simulink model "ABS_fuzzy"  (R2017b)
settings: Solver=VariableStepAuto  StartTime=0.0  StopTime=60  RelTol=1e-3
InitFcn:
  | T_B = 0.1;
  | J = 1.13;
  | g = 9.81;
  | 
  | road_coeff = [
  |                 1.2801 23.990 0.5200
  |                 0.8570 33.822 0.3470
  |                 1.1973 25.168 0.5373
  |                 0.4004 33.708 0.1204
  |                 0.1946 94.129 0.0646
  |                 0.0500 306.39 0.0010
  |               ];
  | load('ANFIS.mat','train_fis');
  | ce = road_coeff(sel,:);
  | run controller_fis
undefined symbols (not defined in the file or in its folder): m, R, v_x
libraries: fuzblock x2, simulink x1
settings Model: Creator=hadlaczkyb  LastModifiedBy=hadlaczkyb

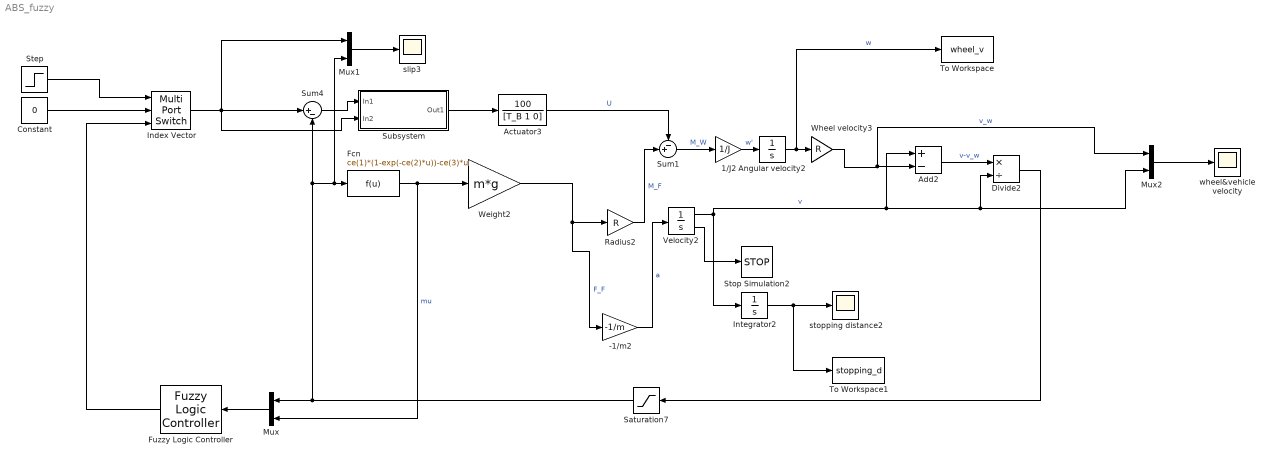
== system ABS_fuzzy ==
  -1/m2 : Gain  Gain=-1/m
  1/J2 : Gain  Gain=1/J
  Actuator3 : TransferFcn  Numerator=[0 0 100]  Denominator=[T_B 1 0]
  Add2 : Sum  Inputs=+-
  Angular velocity2 : Integrator  InitialCondition=v_x/R  LimitOutput=on  UpperSaturationLimit=1000  LowerSaturationLimit=0
  Constant : Constant  Value=0
  Divide2 : Product  Inputs=*/
  Fcn : Fcn  Expr=ce(1)*(1-exp(-ce(2)*u))-ce(3)*u
  Fuzzy Logic Controller : fuzblock/Fuzzy Logic  Controller  FIS=train_fis  OutputSampleNumber=101  DataType=double  FuzzifiedInputs=off  RuleFiringStrengths=off  RuleOutputs=off  AggregatedOutputs=off  SimulateUsing=Interpreted execution
  Index Vector : MultiPortSwitch  DataPortOrder=Zero-based contiguous  Inputs=2  zeroidx=on
  Integrator2 : Integrator
  Mux : Mux  Inputs=2
  Mux1 : Mux  Inputs=2
  Mux2 : Mux  Inputs=2
  Radius2 : Gain  Gain=R
  Saturation7 : Saturate  UpperLimit=1  LowerLimit=0
  Step : Step  Time=5  SampleTime=0
  Stop Simulation2 : Stop
  Subsystem : Subsystem
  Sum1 : Sum  Inputs=-+|
  Sum4 : Sum  Inputs=|+-
  To Workspace : ToWorkspace  VariableName=wheel_v  SaveFormat=Timeseries  SampleTime=-1
  To Workspace1 : ToWorkspace  VariableName=stopping_d  SaveFormat=Timeseries  SampleTime=-1
  Velocity2 : Integrator  InitialCondition=v_x  LimitOutput=on  UpperSaturationLimit=1000  LowerSaturationLimit=1  ShowSaturationPort=on
  Weight2 : Gain  Gain=m*g
  Wheel velocity3 : Gain  Gain=R
  slip3 : Scope
  stopping distance2 : Scope
  wheel&vehicle velocity : Scope
  wires:
  Sum4/1 -> Subsystem/1(In1)
  Mux/1 -> Fuzzy Logic Controller/1
  Saturation7/1 -> Mux1/2, Fcn/1, Sum4/2, Mux/1
  Mux1/1 -> slip3/1
  Fuzzy Logic Controller/1 -> Index Vector/3
  Subsystem/1(Out1) -> Actuator3/1
  Sum1/1 -> 1/J2/1  "M_W"
  -1/m2/1 -> Velocity2/1  "a"
  1/J2/1 -> Angular velocity2/1  "w'"
  Weight2/1 -> -1/m2/1, Radius2/1  "F_F"
  Velocity2/1 -> Integrator2/1, Divide2/2, Mux2/2, Add2/1  "v"
  Integrator2/1 -> To Workspace1/1, stopping distance2/1
  Fcn/1 -> Weight2/1, Mux/2  "mu"
  Divide2/1 -> Saturation7/1
  Radius2/1 -> Sum1/2  "M_F"
  Angular velocity2/1 -> To Workspace/1, Wheel velocity3/1  "w"
  Add2/1 -> Divide2/1  "v-v_w"
  Wheel velocity3/1 -> Add2/2, Mux2/1  "v_w"
  Velocity2/2 -> Stop Simulation2/1
  Actuator3/1 -> Sum1/1  "U"
  Mux2/1 -> wheel&vehicle velocity/1
  Step/1 -> Index Vector/1
  Constant/1 -> Index Vector/2
  Index Vector/1 -> Subsystem/2(In2), Sum4/1, Mux1/1

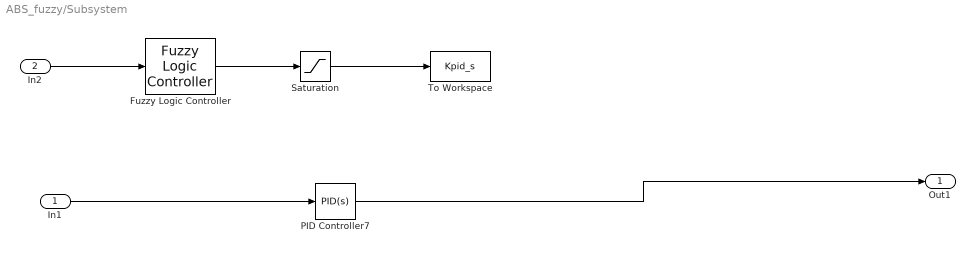
== system ABS_fuzzy/Subsystem ==
  In1 : Inport
  In2 : Inport  Port=2
  Fuzzy Logic Controller : fuzblock/Fuzzy Logic  Controller  FIS=con_fis  OutputSampleNumber=101  DataType=double  FuzzifiedInputs=off  RuleFiringStrengths=off  RuleOutputs=off  AggregatedOutputs=off  SimulateUsing=Interpreted execution
  PID Controller7 : simulink/Continuous/PID Controller  Controller=PID  TimeDomain=Continuous-time  SampleTime=-1  IntegratorMethod=Forward Euler  FilterMethod=Forward Euler  Form=Parallel  UseFilter=on  ControllerParametersSource=internal  P=Kpid_s(end,1)  I=Kpid_s(end,2)  D=Kpid_s(end,3)  N=1000  InitialConditionSource=internal  InitialConditionForIntegrator=0  InitialConditionForFilter=0  ExternalReset=none  LimitOutput=off  UpperSaturationLimit=inf  LowerSaturationLimit=-inf  LinearizeAsGain=on  AntiWindupMode=none  Kb=1  TrackingMode=off  Kt=1  PParamMin=[]  PParamMax=[]  IParamMin=[]  IParamMax=[]  DParamMin=[]  DParamMax=[]  NParamMin=[]  NParamMax=[]  KbParamMin=[]  KbParamMax=[]  KtParamMin=[]  KtParamMax=[]  POutMin=[]  POutMax=[]  IOutMin=[]  IOutMax=[]  DOutMin=[]  DOutMax=[]  NOutMin=[]  NOutMax=[]  KbOutMin=[]  KbOutMax=[]  KtOutMin=[]  KtOutMax=[]  IntegratorOutMin=[]  IntegratorOutMax=[]  FilterOutMin=[]  FilterOutMax=[]  SumOutMin=[]  SumOutMax=[]  SumI1OutMin=[]  SumI1OutMax=[]  SumI2OutMin=[]  SumI2OutMax=[]  SumI3OutMin=[]  SumI3OutMax=[]  SumDOutMin=[]  SumDOutMax=[]  SaturationOutMin=[]  SaturationOutMax=[]  IntegratorContinuousStateAttributes=''  IntegratorStateMustResolveToSignalObject=off  IntegratorRTWStateStorageClass=Auto  FilterContinuousStateAttributes=''  FilterStateMustResolveToSignalObject=off  FilterRTWStateStorageClass=Auto  DifferentiatorICPrevScaledInput=0  DifferentiatorOutMin=[]  DifferentiatorOutMax=[]  InitialConditionSetting=State (most efficient)  FilterDiffOutCoefMin=[]  FilterDiffOutCoefMax=[]  SumDenOutMin=[]  SumDenOutMax=[]  SumNumOutMin=[]  SumNumOutMax=[]  ReciprocalOutMin=[]  ReciprocalOutMax=[]  DivideOutMin=[]  DivideOutMax=[]  TunerSelectOption=Transfer Function Based (PID Tuner App)
  Saturation : Saturate  UpperLimit=1000  LowerLimit=0
  To Workspace : ToWorkspace  VariableName=Kpid_s  SampleTime=-1
  Out1 : Outport  PortDimensions=1
  wires:
  Fuzzy Logic Controller/1 -> Saturation/1
  In2/1 -> Fuzzy Logic Controller/1
  In1/1 -> PID Controller7/1
  PID Controller7/1 -> Out1/1
  Saturation/1 -> To Workspace/1
